simulink model "DFPI_MdlIdent"  (R2017a)
settings: Solver=VariableStepAuto  StartTime=0.0  StopTime=100  FixedStep=0.001  MaxStep=1e-3  RelTol=1e-5  EnableMultiTasking=on
PostLoadFcn:
  | , if any(exist('dsrtsu_mdlpostloadfcn', 'file') == [2, 3, 6]), try dsrtsu_mdlpostloadfcn('Execute', bdroot); catch fprintf('Error in PostLoadFcn (dsrtsu_mdlpostloadfcn) for model "%s":\n %s\n', bdroot, lasterr); end, end,
undefined symbols (not defined in the file or in its folder): mdlPara, PA_models_DFPI, PASL_Models
libraries: PASL_Pneumatics x3, PASL_Components x2, PASL_Tools x2, PASL_Mechanics x1
settings Model: DSRTSU_INTERNAL_RTI_VER=500  DSRTSU_INTERNAL_RTI_TYPE=rti1401  DSRTSU_INTERNAL_RTIFPGA=60  Creator=fbwk  LastModifiedBy=fbwk
settings DataIOCC: LimitDataPoints=on  SaveFormat=Array
settings OptimizationCC: BlockReduction=off  OptimizeBlockIOStorage=off  BufferReuse=off  GlobalBufferReuse=off  ExpressionFolding=off  LocalBlockOutputs=off  LifeSpan=inf
settings DebuggingCC: SolverPrmCheckMsg=warning  SFUnexpectedBacktrackingDiag=warning  SFNoUnconditionalDefaultTransitionDiag=warning  SFExecutionAtInitializationDiag=none
settings HardwareCC: ProdBitPerPointer=32  ProdBitPerSizeT=32  ProdBitPerPtrDiffT=32  ProdLargestAtomicInteger=Integer  ProdEndianess=BigEndian  ProdWordSize=32  ProdHWDeviceType=Custom Processor->Custom  TargetIntDivRoundTo=Zero  TargetEndianess=BigEndian  TargetHWDeviceType=Custom Processor->Custom
settings ModelReferenceCC: PropagateSignalLabelsOutOfModel=off
settings SFSimCC: MATLABDynamicMemAlloc=off
settings RTWCC: SystemTargetFile=rti1005.tlc  MakeCommand=make_rti  TemplateMakefile=rti1005.tmf  Description=dSPACE DS1005 Hardware Platform
settings STFCustomTargetCC: ParMdlRefBuildCompliant=on  MatFileLogging=on  GRTInterface=off  SystemTargetFile=rti1005.tlc
settings GRTTargetCC: TargetLangStandard=C89/C90 (ANSI)  CompOptLevelCompliant=off  ConcurrentExecutionCompliant=off  CombineOutputUpdateFcns=off  CPPClassGenCompliant=off  UseToolchainInfoCompliant=off  ExtModeMexFile=noextcomm
settings ConfigComp: CovMetricSettings=dw  CovHtmlReporting=on  CovSaveCumulativeToWorkspaceVar=on  CovSaveSingleToWorkspaceVar=on  CovExternalEMLEnable=off  CovSFcnEnable=off

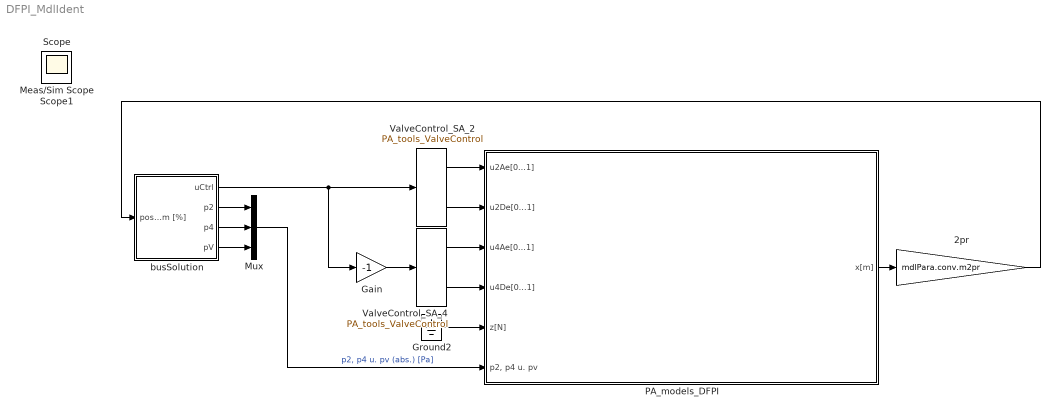
== system DFPI_MdlIdent ==
  2pr : Gain  Gain=mdlPara.conv.m2pr
  Gain : Gain  Gain=-1
  Ground2 : Ground
  Mux : Mux  Inputs=3
  PA_models_DFPI : Subsystem  Tag=PA_models_DFPI  AncestorBlock=PASL_Models/PA_models_DFPI  mask(DFPI Modell){mdlPara=mdlPara}
      mask prompts: mdlPara "Name of the parameters struct:"
      mask help:
      | Dieser Block beinhaltet das DFPI Modell.
      |
      | Zur Initialisierung des Blocks kann entweder
      | a) ein vorhandener Parametersatz geladen werden
      | oder
      | b) ein default Datensatz generiert werden.
      | 	Dabei werden die Daten des DFPI abgefragt
      | 	und alle aus der Konstruktion bekannten
      | 	Parameter entsprechend berechnet.
      | 	Für nicht bekannte Parameter wie z.B.
      | 	Reibung werden default Werte verwendet.
      |
      | 2015-08-28, fbwk
      mask Help: eval(['run(strcat(''',getenv('pasl_simulink'),''',''\documentation\tools\HelpForPaslElements.m''))']);
      mask DialogControl Control2 Prompt: PARAMETERSATZ LADEN
      mask DialogControl Control2 Callback:
      | %% Modellparameter laden %%%%%%%%%%%%%%%%%%%%%%%%%%%%%%%%%%%%%%%%%%%%%%%%%%
      | 
      | % get mask parameters
      | maskval = get_param(gcb,'MaskValues');
      | structName = maskval{1};
      | 
      | % load parameters
      | assignin('base',structName,...
      | 	aux_loadMdlPara('DFPI','mdlPara_DFPI-100-40_08.mat')...
      | 	);
      | 
      | % clear section
      | clear maskval structName
      mask DialogControl Control3 Prompt: default Werte generieren
      mask DialogControl Control3 Callback:
      | %% Modellparameter laden %%%%%%%%%%%%%%%%%%%%%%%%%%%%%%%%%%%%%%%%%%%%%%%%%%
      | 
      | % get mask parameters
      | maskval = get_param(gcb,'MaskValues');
      | structName = maskval{1};
      | 
      | % load parameters
      | assignin('base',structName,aux_initMdlParaDFPI());
      | 
      | % clear section
      | clear maskval structName
      mask Display:
      | image(imread('DFPI_1.jpg'))
      | 
      | port_label('input',3,'u4Ae [0...1]')
      | port_label('input',4,'u4De [0...1]')
      | port_label('input',1,'u2Ae [0...1]')
      | port_label('input',2,'u2De [0...1]')
      | port_label('input',5,'z [N]')
      | 
      | port_label('output',1,'x [m]')
  ValveControl_SA_2 : PASL_Tools/PA_tools_ValveControl
      settings: SourceProductName=PASL
  ValveControl_SA_4 : PASL_Tools/PA_tools_ValveControl
      settings: SourceProductName=PASL
  busSolution : Subsystem  VariantControl=busVariant
  Meas/Sim Scope : Scope
  Scope : Scope
  Scope1 : Scope
  wires:
  ValveControl_SA_2/2 -> PA_models_DFPI/2(u2De[0...1])
  Ground2/1 -> PA_models_DFPI/5(z[N])
  PA_models_DFPI/1(x[m]) -> 2pr/1
  busSolution/2(p2) -> Mux/1
  ValveControl_SA_2/1 -> PA_models_DFPI/1(u2Ae[0...1])
  2pr/1 -> busSolution/1(posSim [%])
  ValveControl_SA_4/1 -> PA_models_DFPI/3(u4Ae[0...1])
  ValveControl_SA_4/2 -> PA_models_DFPI/4(u4De[0...1])
  Gain/1 -> ValveControl_SA_4/1
  busSolution/3(p4) -> Mux/2
  Mux/1 -> PA_models_DFPI/6("p2, p4 u. pv")  "p2, p4 u. pv (abs.) [Pa]"
  busSolution/4(pV) -> Mux/3
  busSolution/1(uCtrl) -> ValveControl_SA_2/1, Gain/1

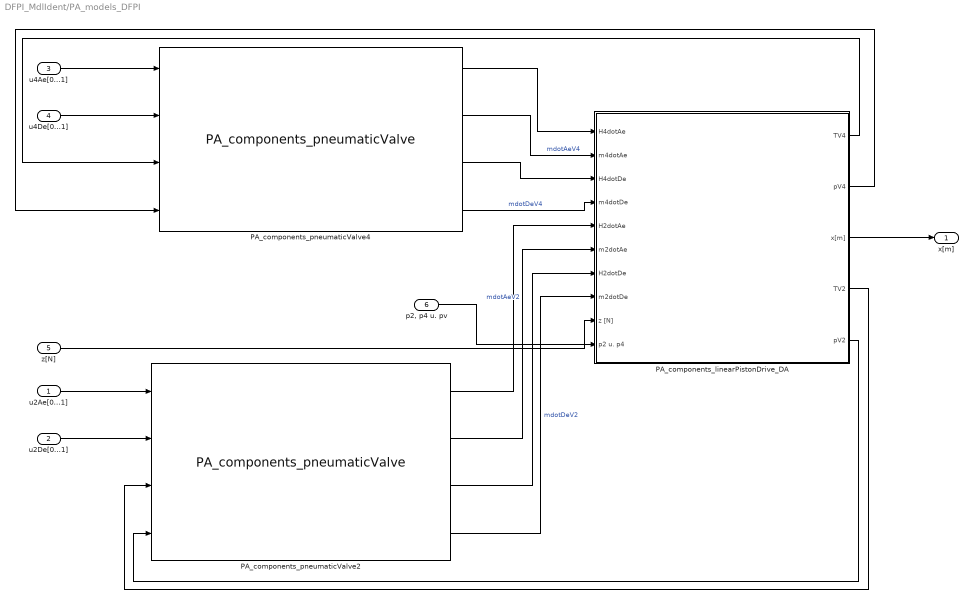
== system DFPI_MdlIdent/PA_models_DFPI ==
  u2Ae[0...1] : Inport
  u2De[0...1] : Inport  Port=2
  u4Ae[0...1] : Inport  Port=3
  u4De[0...1] : Inport  Port=4
  z[N] : Inport  Port=5
  "p2, p4 u. pv" : Inport  Port=6
  PA_components_linearPistonDrive_DA : Subsystem  AncestorBlock=PASL_Components/PA_components_linearPistonDrive_DA  mask(Linear Piston Drive Double Acting){p02=mdlPara.p02, p04=mdlPara.p04, T0=mdlPara.Tu, V02=mdlPara.V02, V04=mdlPara.V04, heatExCoeff=mdlPara.heatExCoeff, Tu=mdlPara.Tu, heatExArea=mdlPara.heatExArea, R=mdlPara.R, n=mdlPara.n, smoothFac=mdlPara.smoothFac, d2Out=mdlPara.d2Out, d2In=mdlPara.d2In, d4Out=mdlPara.d4Out, d4In=mdlPara.d4In, pu=mdlPara.pu, x0=mdlPara.x0, x02=mdlPara.x02, x04=mdlPara.x04, Fl=mdlPara.Fl, v0=mdlPara.v0, mass=mdlPara.mass, viscFriCoeff1=mdlPara.viscFriCoeff1, viscFriCoeff2=mdlPara.viscFriCoeff2, viscFriCoeff3=mdlPara.viscFriCoeff3, stribeckVel=mdlPara.stribeckVel, Fstick=mdlPara.Fstick, Fcoulomb=mdlPara.Fcoulomb, xMin=mdlPara.xMin, xMax=mdlPara.xMax}
      mask prompts: p02 "Initial pressure volume 2 [pa]"; p04 "Initial pressure volume 4 [pa]"; T0 "Initial temperature[k]"; V02 "Initial volume 2[m^3]"; V04 "Initial volume 4[m^3]"; heatExCoeff "Heat exchange coefficent [J/(s*m^2*K)]"; Tu "Wall temperature [K]"; heatExArea "Heat exchange area"; R "Gas constant [J/(kg*K)]"; n "Polytropic exponent [1]"; smoothFac "Smooth Factor [1]"; d2Out "Outer diameter volume 2 [m]"; d2In "Inner diameter volume [m]"; d4Out "Outer diameter volume 4 [m]"; d4In "Inner diameter volume 4 [m]"; pu "Ambient pressure [Pa]"; x0 "Initial displacement [m]"; x02 "Initial length Chamber 2 [m]"; x04 "Initial length Chamber 4 [m]"; Fl "Force fluid [N]"; v0 "Initial velocity [m/s]"; mass "Mass [kg]"; viscFriCoeff1 "Coeff. 1 for viscous friction [Ns/m]"; viscFriCoeff2 "Coeff. 2 viscous friction [Ns^2/m^2]"; viscFriCoeff3 "Coeff. 3 for viscous friction [Ns^3/m^3]"; stribeckVel "Stribeck velocity [m/s]"; Fstick "Force at stick Friction (FStick) [N]"; Fcoulomb "Force at Coulomb friction < Fstick [N]"; xMin "Lower displacement limit (xmin) [m]"; xMax "Upper displacement limit > xmin [m]"
      mask help:
      | DESCRIPTION : Festo Process Automation Library Standard Element.
      |
      | This is a model of a double acting linear piston drive.
      |
      | ------------------------------------------------------------------------------
      | INPUTS:
      | H4dotAe	- Enthalpy flow (Aeration) Chamber 4            [J/s]
      | m4dotAe	- Mass flow (Aeration) Chamber 4                [kg/s]
      | H4dotDe	- Enthalpy flow (Deaeration) Chamber 4         [J/s]
      | m4dotDe	- Mass flow (Deaeration) Chamber 4             [kg/s]
      | H2dotAe	- Enthalpy flow (Aeration) Chamber 2            [J/s]
      | m2dotAe	- Mass flow (Aeration) Chamber 2                 [kg/s]
      | H2dotDe	- Enthalpy flow (Deaeration) Chamber 2         [J/s]
      | m2dotDe	- Mass flow (Deaeration) Chamber 2             [kg/s]
      | z                  - Disturbance                                               [F]
      |
      | OUTPUTS:
      | TV4	- Chamber temperature in Chamber 4             [K]
      | pV4	- Chamber pressure in Chamber 4                  [Pa]
      | x	- Piston displacement                                     [m]
      | TV2	- Chamber temperature in Chamber 2             [K]
      | pV2	- Chamber pressure in Chamber 2                  [Pa]
      |
      |
      | cdr, 03.05.17
      mask Help: eval(['run(strcat(''',getenv('pasl_simulink'),''',''\documentation\tools\HelpForPaslElements.m''))']);
      mask Display:
      | image(imread('PA_components_DFPK_DA.jpg'));
      | 
      | port_label('input',1, 'H4dotAe [J/s]');
      | port_label('input',2, 'm4dotAe [kg/s]');
      | port_label('input',3, 'H4dotDe [J/s]');
      | port_label('input',4, 'm4dotDe [kg/s]');
      | port_label('input',5, 'H2dotAe [J/s]');
      | port_label('input',6, 'm2dotAe [kg/s]');
      | port_label('input',7, 'H2dotDe [J/s]');
      | port_label('input',8, 'm2dotDe [kg/s]');
      | port_label('input',9, 'z [N]');
      | 
      | port_label('output',1, 'TV4 [K]');
      | port_label('output',2, 'pV4 [Pa]');
      | port_label('output',3, 'x [m]');
      | port_label('output',4, 'TV2 [K]');
      | port_label('output',5, 'pV2 [Pa]');
  PA_components_pneumaticValve2 : PASL_Components/PA_components_pneumaticValve  b=mdlPara.b  C=mdlPara.C2  pv=mdlPara.pv  pu=mdlPara.pu  Tu=mdlPara.Tu  R=mdlPara.R  n=mdlPara.n  smoothFact=mdlPara.smoothFac
      settings: SourceProductName=PASL
  PA_components_pneumaticValve4 : PASL_Components/PA_components_pneumaticValve  b=mdlPara.b  C=mdlPara.C4  pv=mdlPara.pv  pu=mdlPara.pu  Tu=mdlPara.Tu  R=mdlPara.R  n=mdlPara.n  smoothFact=mdlPara.smoothFac
      settings: SourceProductName=PASL
  x[m] : Outport
  wires:
  u4Ae[0...1]/1 -> PA_components_pneumaticValve4/1
  PA_components_linearPistonDrive_DA/4(TV2) -> PA_components_pneumaticValve2/3
  PA_components_linearPistonDrive_DA/5(pV2) -> PA_components_pneumaticValve2/4
  PA_components_pneumaticValve2/1 -> PA_components_linearPistonDrive_DA/5(H2dotAe)
  PA_components_pneumaticValve4/3 -> PA_components_linearPistonDrive_DA/3(H4dotDe)
  PA_components_pneumaticValve2/4 -> PA_components_linearPistonDrive_DA/8(m2dotDe)  "mdotDeV2"
  u2De[0...1]/1 -> PA_components_pneumaticValve2/2
  PA_components_pneumaticValve2/3 -> PA_components_linearPistonDrive_DA/7(H2dotDe)
  u4De[0...1]/1 -> PA_components_pneumaticValve4/2
  PA_components_pneumaticValve2/2 -> PA_components_linearPistonDrive_DA/6(m2dotAe)  "mdotAeV2"
  PA_components_pneumaticValve4/4 -> PA_components_linearPistonDrive_DA/4(m4dotDe)  "mdotDeV4"
  PA_components_linearPistonDrive_DA/2(pV4) -> PA_components_pneumaticValve4/4
  PA_components_pneumaticValve4/2 -> PA_components_linearPistonDrive_DA/2(m4dotAe)  "mdotAeV4"
  PA_components_linearPistonDrive_DA/3(x[m]) -> x[m]/1
  u2Ae[0...1]/1 -> PA_components_pneumaticValve2/1
  PA_components_pneumaticValve4/1 -> PA_components_linearPistonDrive_DA/1(H4dotAe)
  z[N]/1 -> PA_components_linearPistonDrive_DA/9(z [N])
  PA_components_linearPistonDrive_DA/1(TV4) -> PA_components_pneumaticValve4/3
  "p2, p4 u. pv"/1 -> PA_components_linearPistonDrive_DA/10(p2 u. p4)

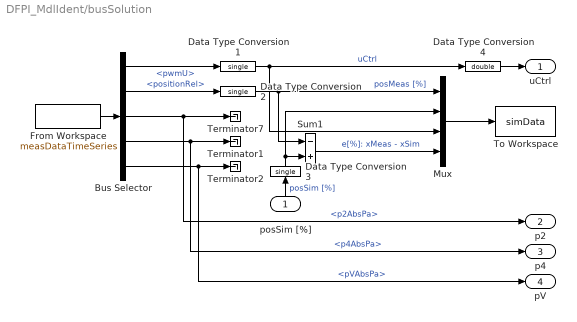
== system DFPI_MdlIdent/busSolution ==
  posSim [%] : Inport
  Bus Selector : BusSelector  OutputSignals=pwmU,positionRel,p2AbsPa,p4AbsPa,pVAbsPa
  Data Type Conversion1 : DataTypeConversion  OutDataTypeStr=single
  Data Type Conversion2 : DataTypeConversion  OutDataTypeStr=single
  Data Type Conversion3 : DataTypeConversion  OutDataTypeStr=single
  Data Type Conversion4 : DataTypeConversion  OutDataTypeStr=double
  From Workspace : FromWorkspace  VariableName=measDataTimeSeries  OutDataTypeStr=Bus: busMeasData  SampleTime=0
  Mux : Mux
  Sum1 : Sum  Inputs=-+
  Terminator1 : Terminator
  Terminator2 : Terminator
  Terminator7 : Terminator
  To Workspace : ToWorkspace  VariableName=simData  SaveFormat=Structure With Time  SampleTime=-1
  uCtrl : Outport
  p2 : Outport  Port=2
  p4 : Outport  Port=3
  pV : Outport  Port=4
  wires:
  Data Type Conversion4/1 -> uCtrl/1
  Data Type Conversion3/1 -> Mux/2, Sum1/2
  Data Type Conversion2/1 -> Mux/1, Sum1/1  "posMeas [%]"
  Data Type Conversion1/1 -> Data Type Conversion4/1, Mux/3  "uCtrl"
  Mux/1 -> To Workspace/1
  Sum1/1 -> Mux/4  "e[%]: xMeas - xSim"
  posSim [%]/1 -> Data Type Conversion3/1  "posSim [%]"
  Bus Selector/3 -> Terminator7/1, p2/1  "<p2AbsPa>"
  From Workspace/1 -> Bus Selector/1
  Bus Selector/4 -> Terminator1/1, p4/1  "<p4AbsPa>"
  Bus Selector/2 -> Data Type Conversion2/1  "<positionRel>"
  Bus Selector/1 -> Data Type Conversion1/1  "<pwmU>"
  Bus Selector/5 -> Terminator2/1, pV/1  "<pVAbsPa>"

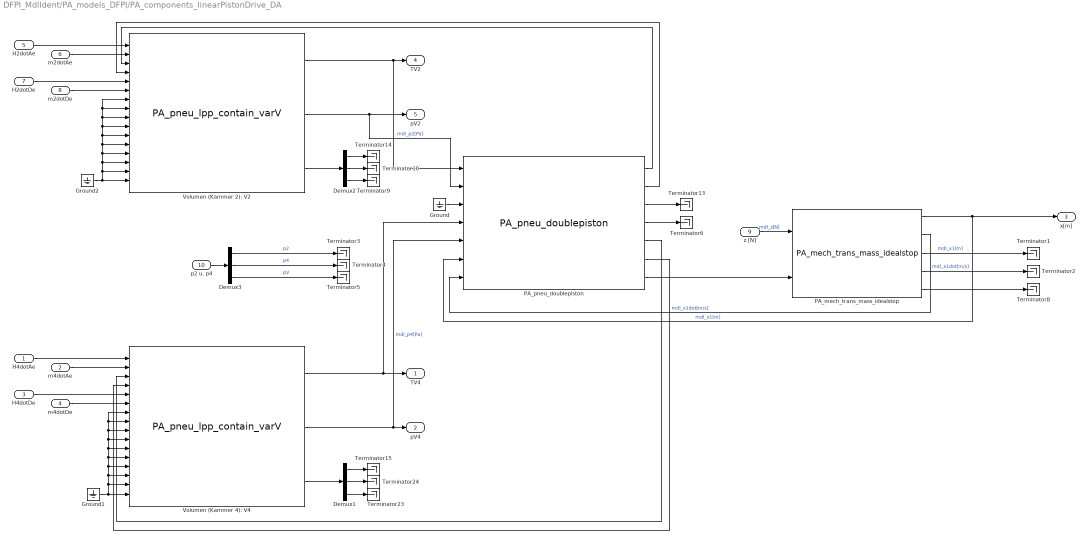
== system DFPI_MdlIdent/PA_models_DFPI/PA_components_linearPistonDrive_DA ==
  H4dotAe : Inport
  m4dotAe : Inport  Port=2
  H4dotDe : Inport  Port=3
  m4dotDe : Inport  Port=4
  H2dotAe : Inport  Port=5
  m2dotAe : Inport  Port=6
  H2dotDe : Inport  Port=7
  m2dotDe : Inport  Port=8
  z [N] : Inport  Port=9
  p2 u. p4 : Inport  Port=10
  Demux1 : Demux  Outputs=3
  Demux2 : Demux  Outputs=3
  Demux3 : Demux  Outputs=3
  Ground : Ground
  Ground1 : Ground
  Ground2 : Ground
  PA_mech_trans_mass_idealstop : PASL_Mechanics/Moving Masses/PA_mech_trans_mass_idealstop  Tag=RB_mech_trans_mass_idealstop  xinit=x0  xdotinit=v0  m=mass  dtrans1=viscFriCoeff1  dtrans2=viscFriCoeff2  dtrans3=viscFriCoeff3  xdotstri=stribeckVel  Fstick=Fstick  Fslip=Fcoulomb  xmin=xMin  xmax=xMax
      settings: SourceProductName=PASL
  PA_pneu_doublepiston : PASL_Pneumatics/Pistons/PA_pneu_doublepiston  d_out2=d2Out  d_in2=d2In  d_out4=d4Out  d_in4=d4In  x_02=x02  x_04=x04  p0=pu
      settings: SourceProductName=PASL
  Terminator{1..6,8..10,13..15,23..24} (14 alike) : Terminator
  Volumen (Kammer 2): V2 : PASL_Pneumatics/Volumes/PA_pneu_lpp_contain_varV  p0=p02  T0=Tu  V0=V02  K=heatExCoeff  A=heatExArea  Tw=Tu  R=R  kappa=n  temp_effects=without temperature effects
      settings: SourceProductName=PASL
  Volumen (Kammer 4): V4 : PASL_Pneumatics/Volumes/PA_pneu_lpp_contain_varV  p0=p04  T0=Tu  V0=V04  K=heatExCoeff  A=heatExArea  Tw=Tu  R=R  kappa=n  temp_effects=without temperature effects
      settings: SourceProductName=PASL
  TV4 : Outport
  pV4 : Outport  Port=2
  x[m] : Outport  Port=3
  TV2 : Outport  Port=4
  pV2 : Outport  Port=5
  wires:
  PA_mech_trans_mass_idealstop/4 -> Terminator2/1  "mdl_x1dot[m/s]"
  PA_mech_trans_mass_idealstop/3 -> Terminator1/1  "mdl_x1[m]"
  H4dotDe/1 -> Volumen (Kammer 4): V4/5
  m4dotDe/1 -> Volumen (Kammer 4): V4/6
  m4dotAe/1 -> Volumen (Kammer 4): V4/2
  H4dotAe/1 -> Volumen (Kammer 4): V4/1
  H2dotDe/1 -> Volumen (Kammer 2): V2/5
  m2dotDe/1 -> Volumen (Kammer 2): V2/6
  m2dotAe/1 -> Volumen (Kammer 2): V2/2
  H2dotAe/1 -> Volumen (Kammer 2): V2/1
  z [N]/1 -> PA_mech_trans_mass_idealstop/1  "mdl_z[N]"
  Volumen (Kammer 4): V4/1 -> PA_pneu_doublepiston/4, TV4/1
  Volumen (Kammer 4): V4/2 -> PA_pneu_doublepiston/5, pV4/1  "mdl_p4[Pa]"
  Ground1/1 -> Volumen (Kammer 4): V4/16, Volumen (Kammer 4): V4/15, Volumen (Kammer 4): V4/14, Volumen (Kammer 4): V4/13, Volumen (Kammer 4): V4/12, Volumen (Kammer 4): V4/11, Volumen (Kammer 4): V4/8, Volumen (Kammer 4): V4/7, Volumen (Kammer 4): V4/9, Volumen (Kammer 4): V4/10
  Volumen (Kammer 2): V2/1 -> PA_pneu_doublepiston/1, TV2/1
  Volumen (Kammer 2): V2/2 -> PA_pneu_doublepiston/2, pV2/1  "mdl_p2[Pa]"
  Ground2/1 -> Volumen (Kammer 2): V2/15, Volumen (Kammer 2): V2/14, Volumen (Kammer 2): V2/13, Volumen (Kammer 2): V2/12, Volumen (Kammer 2): V2/11, Volumen (Kammer 2): V2/8, Volumen (Kammer 2): V2/7, Volumen (Kammer 2): V2/9, Volumen (Kammer 2): V2/10, Volumen (Kammer 2): V2/16
  PA_mech_trans_mass_idealstop/2 -> PA_pneu_doublepiston/7  "mdl_x1dot[m/s]"
  Volumen (Kammer 4): V4/3 -> Demux1/1
  Demux1/1 -> Terminator15/1
  Volumen (Kammer 2): V2/3 -> Demux2/1
  Demux2/1 -> Terminator14/1
  Demux2/2 -> Terminator10/1
  Demux2/3 -> Terminator9/1
  Demux1/2 -> Terminator24/1
  Demux1/3 -> Terminator23/1
  PA_pneu_doublepiston/3 -> Terminator13/1
  PA_pneu_doublepiston/4 -> Terminator6/1
  PA_mech_trans_mass_idealstop/1 -> PA_pneu_doublepiston/6, x[m]/1  "mdl_x1[m]"
  PA_mech_trans_mass_idealstop/5 -> Terminator8/1
  Ground/1 -> PA_pneu_doublepiston/3
  PA_pneu_doublepiston/7 -> PA_mech_trans_mass_idealstop/2
  PA_pneu_doublepiston/1 -> Volumen (Kammer 2): V2/3
  PA_pneu_doublepiston/2 -> Volumen (Kammer 2): V2/4
  PA_pneu_doublepiston/6 -> Volumen (Kammer 4): V4/4
  PA_pneu_doublepiston/5 -> Volumen (Kammer 4): V4/3
  Demux3/1 -> Terminator3/1  "p2"
  Demux3/3 -> Terminator5/1  "pV"
  Demux3/2 -> Terminator4/1  "p4"
  p2 u. p4/1 -> Demux3/1
